simulink model "MidSideProcessor_Start"  (R2026a)
settings: Solver=FixedStepDiscrete  StopTime=10
libraries: MyMidSideLibrary x2, dspsnks4 x1, dspvision x1
settings Model: Creator=Adam
settings DebuggingCC: AlgebraicLoopMsg=error  SingleTaskRateTransMsg=error

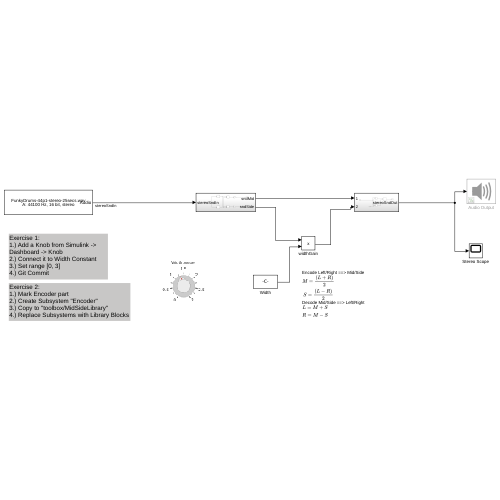
[thumbnail: Simulink's stored preview of the top-level diagram]
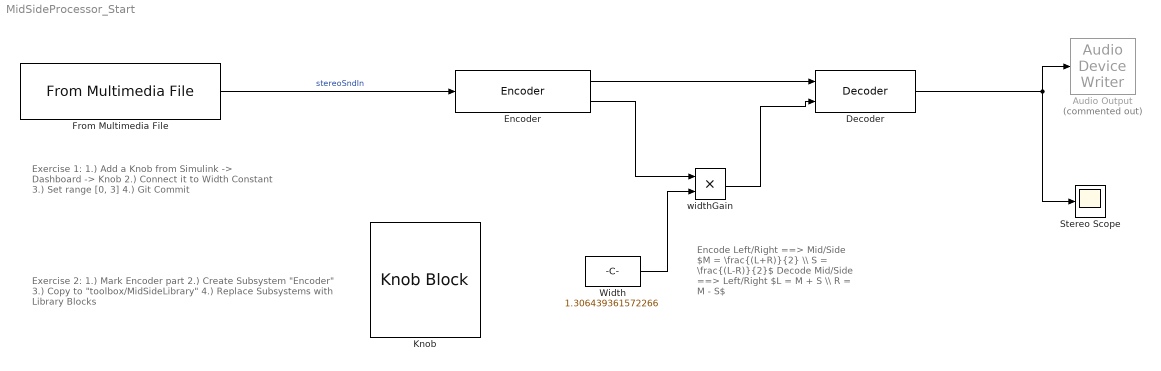
== system MidSideProcessor_Start ==
  note: Exercise 1:
      | 1.) Add a Knob from Simulink -> Dashboard -> Knob
      | 2.) Connect it to Width Constant
      | 3.) Set range [0, 3]
      | 4.) Git Commit
  note: Encode Left/Right ==> Mid/Side
      | $M = \frac{(L+R)}{2} \\ S = \frac{(L-R)}{2}$
      | Decode Mid/Side ==> Left/Right
      | $L = M + S \\ R = M - S$
  note: Exercise 2:
      | 1.) Mark Encoder part
      | 2.) Create Subsystem "Encoder"
      | 3.) Copy to "toolbox/MidSideLibrary"
      | 4.) Replace Subsystems with Library Blocks
  Audio Output : dspsnks4/Audio Device Writer  Commented=on  Driver=ALSA  Device=No audio output device detected  InheritSampleRate=on  SampleRate=44100  BitDepth=16-bit integer  BufferSize=4096  NumBuffers=10  DefaultOutputChannelMapping=on  OutputChannelMapping=1:2  OutputNumUnderrunSamples=off  DriverIdx=8  DeviceWarnFlag=''
  Decoder : MyMidSideLibrary/Decoder  SystemSampleTime=-1  VariantActivationTime=update diagram  EmptyChoice=off  PassThrough=off  PassThroughVariantControl=(default)  EmptyChoiceVariantControl=(default)  AllowFlexibleInterface=on  Latency=0  AutoFrameSizeCalculation=off
  Encoder : MyMidSideLibrary/Encoder  SystemSampleTime=-1  VariantActivationTime=update diagram  EmptyChoice=off  PassThrough=off  PassThroughVariantControl=(default)  EmptyChoiceVariantControl=(default)  AllowFlexibleInterface=on  Latency=0  AutoFrameSizeCalculation=off
  From Multimedia File : dspvision/From Multimedia File  inputFilename=FunkyDrums-44p1-stereo-25secs.wav  readRange=[1 Inf]  loop=on  numPlays=inf  outputStreams=Audio only  videoDataType=single  audioDataType=double  inheritSampleTime=on  userDefinedSampleTime=1/30  noAudioOutput=off  isIntensityVideo=off  fourcc=RGB  colorVideoFormat=Separate color signals  outputEOF=off  dataOrg=Column-major  audioFrameSize=1024  computeAudioFrameSize=off  outSamplingMode=Sample based
  Knob : KnobBlock  ScaleMax=3
  Stereo Scope : Scope
      settings: TimeUnits=Metric (based on Time Span)  ActiveDisplayYMinimum=-0.86994171142578125  ActiveDisplayYMaximum=1.0567092895507812  YLabel=Amplitude
  Width : Constant  Value=1.306439361572266
  widthGain : Product
  wires:
  Width/1 -> widthGain/2
  From Multimedia File/1 -> Encoder/1  "stereoSndIn"
  Encoder/2 -> widthGain/1
  Decoder/1 -> Stereo Scope/1, Audio Output/1
  Encoder/1 -> Decoder/1
  widthGain/1 -> Decoder/2
